simulink model "algLoopRemodel"  (R2022b)
settings: Solver=ode45  StartTime=0.0  StopTime=10.0  RelTol=1e-3  EnableMultiTasking=on
settings Model: Creator=jrivitus  LastModifiedBy=bensweet
settings SolverCC: AlgebraicLoopSolver=TrustRegion
settings DataIOCC: LimitDataPoints=on  SaveFormat=Array  ReturnWorkspaceOutputs=off
settings OptimizationCC: ExpressionDepthLimit=2147483647  LifeSpan=inf
settings DebuggingCC: UnconnectedInputMsg=warning  UnconnectedOutputMsg=warning  UnconnectedLineMsg=warning  PregeneratedLibrarySubsystemCodeDiagnostic=none  SFMachineParentedDataDiag=warning
settings HardwareCC: ProdBitPerPointer=32  ProdBitPerSizeT=32  ProdBitPerPtrDiffT=32  ProdLargestAtomicFloat=None  ProdIntDivRoundTo=Undefined  ProdEndianess=Unspecified  ProdWordSize=32  ProdHWDeviceType=32-bit Generic
settings ModelReferenceCC: EnableRefExpFcnMdlSchedulingChecks=on  PropagateSignalLabelsOutOfModel=off
settings SFSimCC: SimUseLocalCustomCode=off
settings RTWCC: RTWUseLocalCustomCode=off  DLArmComputeVersion=19.05
settings CodeAppCC: StateflowObjectComments=on
settings GRTTargetCC: TargetLangStandard=C89/C90 (ANSI)  CombineOutputUpdateFcns=off  GRTInterface=on
settings ConfigComp: CovMetricSettings=dw  CovSaveCumulativeToWorkspaceVar=on  CovSaveSingleToWorkspaceVar=on  CovExternalEMLEnable=off  CovSFcnEnable=off

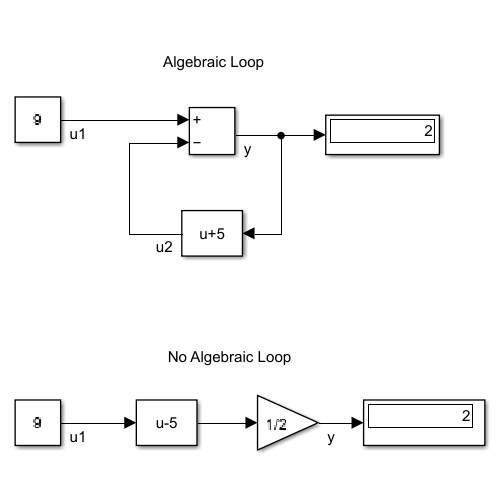
[thumbnail: Simulink's stored preview of the top-level diagram]
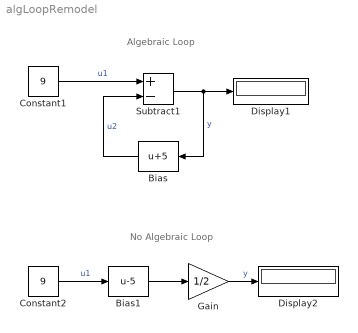
== system algLoopRemodel ==
  note: Algebraic Loop
  note: No Algebraic Loop
  Bias : Bias  Bias=5  SaturateOnIntegerOverflow=off
  Bias1 : Bias  Bias=-5  SaturateOnIntegerOverflow=off
  Constant1 : Constant  Value=9
  Constant2 : Constant  Value=9
  Display1 : Display
  Display2 : Display
  Gain : Gain  Gain=1/2
  Subtract1 : Sum  Inputs=+-
  wires:
  Bias/1 -> Subtract1/2  "u2"
  Constant1/1 -> Subtract1/1  "u1"
  Subtract1/1 -> Display1/1, Bias/1  "y"
  Constant2/1 -> Bias1/1  "u1"
  Bias1/1 -> Gain/1
  Gain/1 -> Display2/1  "y"
